simulink model "Ej4"  (R2016a)
settings: Solver=ode45  StartTime=0.0  StopTime=10.0  RelTol=1e-3
settings Model: Creator=masar_000  LastModifiedBy=Abel
settings DataIOCC: LimitDataPoints=on  SaveFormat=Array
settings DebuggingCC: SolverPrmCheckMsg=warning
settings HardwareCC: ProdBitPerPointer=32  ProdLargestAtomicFloat=None  ProdIntDivRoundTo=Undefined  ProdEndianess=Unspecified  ProdWordSize=32  ProdHWDeviceType=32-bit Generic
settings ModelReferenceCC: PropagateSignalLabelsOutOfModel=off
settings ConfigComp: CovModelRefEnable=Off  CovSFcnEnable=off

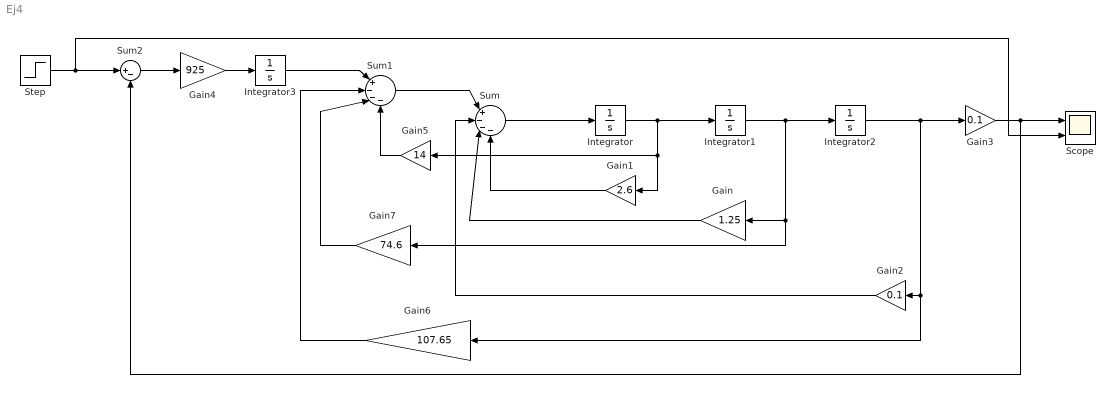
== system Ej4 ==
  Gain : Gain  Gain=1.25
  Gain1 : Gain  Gain=2.6
  Gain2 : Gain  Gain=0.1
  Gain3 : Gain  Gain=0.1
  Gain4 : Gain  Gain=925
  Gain5 : Gain  Gain=14
  Gain6 : Gain  Gain=107.65
  Gain7 : Gain  Gain=74.6
  Integrator{,1..3} (4 alike) : Integrator
  Scope : Scope  NumInputPorts=2
  Step : Step  SampleTime=0
  Sum : Sum  Inputs=|+---
  Sum1 : Sum  Inputs=|+---
  Sum2 : Sum  Inputs=|+-
  wires:
  Sum/1 -> Integrator/1
  Integrator/1 -> Gain5/1, Gain1/1, Integrator1/1
  Integrator1/1 -> Gain7/1, Gain/1, Integrator2/1
  Gain1/1 -> Sum/4
  Gain/1 -> Sum/3
  Integrator2/1 -> Gain6/1, Gain2/1, Gain3/1
  Gain2/1 -> Sum/2
  Gain5/1 -> Sum1/4
  Gain7/1 -> Sum1/3
  Gain6/1 -> Sum1/2
  Integrator3/1 -> Sum1/1
  Sum2/1 -> Gain4/1
  Gain4/1 -> Integrator3/1
  Gain3/1 -> Sum2/2, Scope/1
  Step/1 -> Scope/2, Sum2/1
  Sum1/1 -> Sum/1
